simulink model "lab_3"  (R2024a)
settings: Solver=ode4  StartTime=0.0  StopTime=100.0  FixedStep=0.01  RelTol=1e-3
settings Model: Creator=lw53894  LastModifiedBy=lw53894

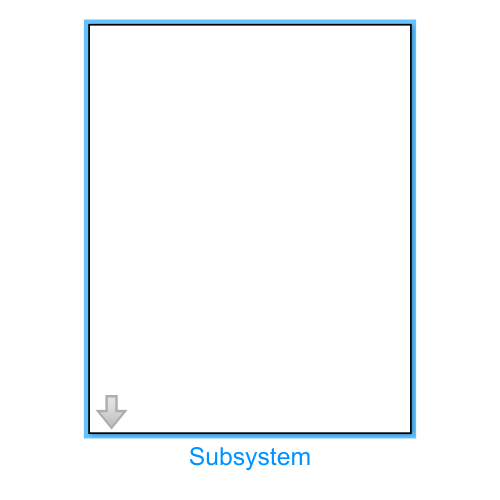
[thumbnail: Simulink's stored preview of the top-level diagram]
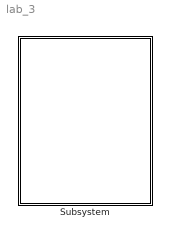
== system lab_3 ==
  Subsystem : Subsystem  mask{k=1, m=10, g=10, l=3, x=90}
      mask prompts: k "wsp. tłumienia"; m "masa wahadła"; g "przyśpieszenie ziemskie"; l "długość wahadła"; x "kąt wychylenia wahadła"

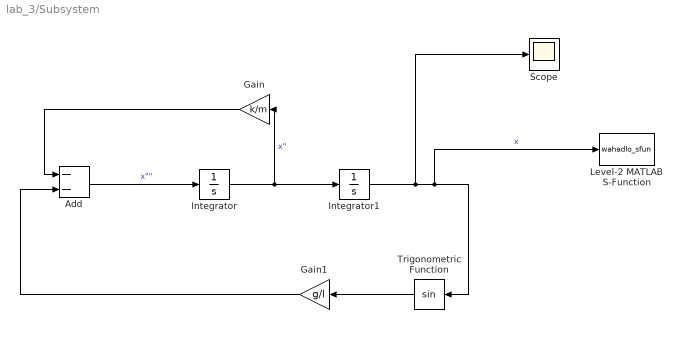
== system lab_3/Subsystem ==
  Add : Sum  Inputs=--
  Gain : Gain  Gain=k/m
  Gain1 : Gain  Gain=g/l
  Integrator : Integrator
  Integrator1 : Integrator  InitialCondition=(x*pi)/180
  Level-2 MATLAB S-Function : M-S-Function  FunctionName=wahadlo_sfun  Parameters=l,m,x
  Scope : Scope
  Trigonometric Function : Trigonometry
  wires:
  Integrator1/1 -> Level-2 MATLAB S-Function/1, Trigonometric Function/1, Scope/1  "x"
  Gain1/1 -> Add/2
  Integrator/1 -> Gain/1, Integrator1/1  "x\""
  Gain/1 -> Add/1
  Add/1 -> Integrator/1  "x\"\""
  Trigonometric Function/1 -> Gain1/1
